simulink model "ME425QuadcoptorMotionControlV2"  (R2024b)
settings: Solver=VariableStepAuto  StartTime=0.0  StopTime=simTime  FixedStep=0.0001  RelTol=1e-2
undefined symbols (not defined in the file): D_phi, D_psi, D_theta, D_z, g, I_phi, I_psi, I_theta, I_z, initialAngles, Ix, Iy, Iz, m, P__phi, P_psi, P_theta, P_z, zDesired
settings Model: Creator=Arda Gencer  LastModifiedBy=Arda Gencer

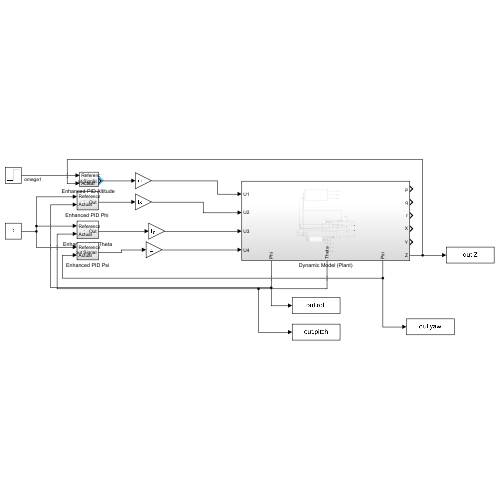
[thumbnail: Simulink's stored preview of the top-level diagram]
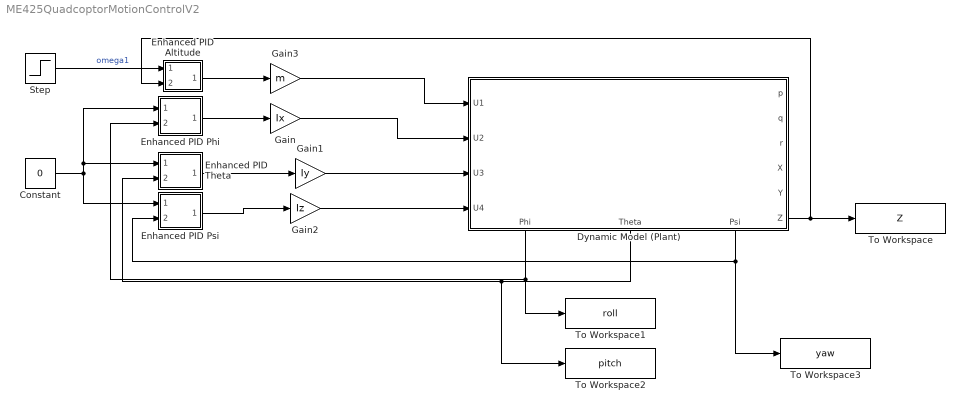
== system ME425QuadcoptorMotionControlV2 ==
  Constant : Constant  Value=0
  Dynamic Model (Plant) : Subsystem
      settings: PortSchema="{\"entries\":[{\"content\":{\"sides\":[{\"content\":{\"connectorIds\":[\"In1\",\"In2\",\"In3\",\"In4\"]},\"type\":\"ConnectorPlacement.EquallySpacedRectSide\",\"uuid\":\"08b1677c-733e-4bff-a275-c4be774b24b5\"},{\"content\":{\"connectorIds\":[\"Out1\",\"Out2\",\"Out3\",\"Out4\",\"Out5\",\"Out6\"],\"side\":\"RIGHT\"},\"type\":\"ConnectorPlacement.EquallySpacedRectSide\",\"uuid\":\"655169e1-9348-4dc0-9050-0d096e576661\"},{\"content\":{\"side\":\"TOP\"},\"type\":\"ConnectorPlacement.EquallySpacedRectSide\",\"uuid\":\"6c01dbd3-88d9-43d1-9966-b2f3dc36f972\"},{\"content\":{\"connectorIds\":[\"Out7\",\"Out8\",\"Out9\"],\"side\":\"BOTTOM\"},\"type\":\"ConnectorPlacement.EquallySpacedRectSide\",\"uuid\":\"d00d5ad9-d72f-434d-885b-77b5f35ca427\"}]},\"type\":\"ConnectorPlacement.EquallySpacedConnector\",\"uuid\":\"87e83324-135b-4426-b2c1-a0cfdb552e41\"}],\"packageUris\":[\"http://schema.mathworks.com/mf0/Connector/R2020b\"],\"version\":\"1.0\"}"
  "Enhanced PID Altitude " : Subsystem
  "Enhanced PID Phi " : Subsystem
  Enhanced PID Psi : Subsystem
  Enhanced PID Theta : Subsystem
  Gain : Gain  Gain=Ix
  Gain1 : Gain  Gain=Iy
  Gain2 : Gain  Gain=Iz
  Gain3 : Gain  Gain=m
  Step : Step  Time=0  After=zDesired  SampleTime=0
  To Workspace : ToWorkspace  VariableName=Z  SampleTime=-1
  To Workspace1 : ToWorkspace  VariableName=roll  SampleTime=-1
  To Workspace2 : ToWorkspace  VariableName=pitch  SampleTime=-1
  To Workspace3 : ToWorkspace  VariableName=yaw  SampleTime=-1
  wires:
  "Enhanced PID Phi "/1(Out) -> Gain/1
  Gain/1 -> Dynamic Model (Plant)/2(U2)
  Gain1/1 -> Dynamic Model (Plant)/3(U3)
  Enhanced PID Theta/1(Out) -> Gain1/1
  Enhanced PID Psi/1(Output Signal) -> Gain2/1
  Gain2/1 -> Dynamic Model (Plant)/4(U4)
  "Enhanced PID Altitude "/1(Output Signal) -> Gain3/1
  Gain3/1 -> Dynamic Model (Plant)/1(U1)
  Dynamic Model (Plant)/6(Z) -> "Enhanced PID Altitude "/2(Actual), To Workspace/1
  Dynamic Model (Plant)/7(Phi) -> To Workspace1/1, "Enhanced PID Phi "/2(Actual)
  Dynamic Model (Plant)/8(Theta) -> To Workspace2/1, Enhanced PID Theta/2(Actual)
  Dynamic Model (Plant)/9(Psi) -> To Workspace3/1, Enhanced PID Psi/2(Actual)
  Constant/1 -> Enhanced PID Psi/1(Reference), Enhanced PID Theta/1(Reference), "Enhanced PID Phi "/1(Reference)
  Step/1 -> "Enhanced PID Altitude "/1(Reference)  "omega1"

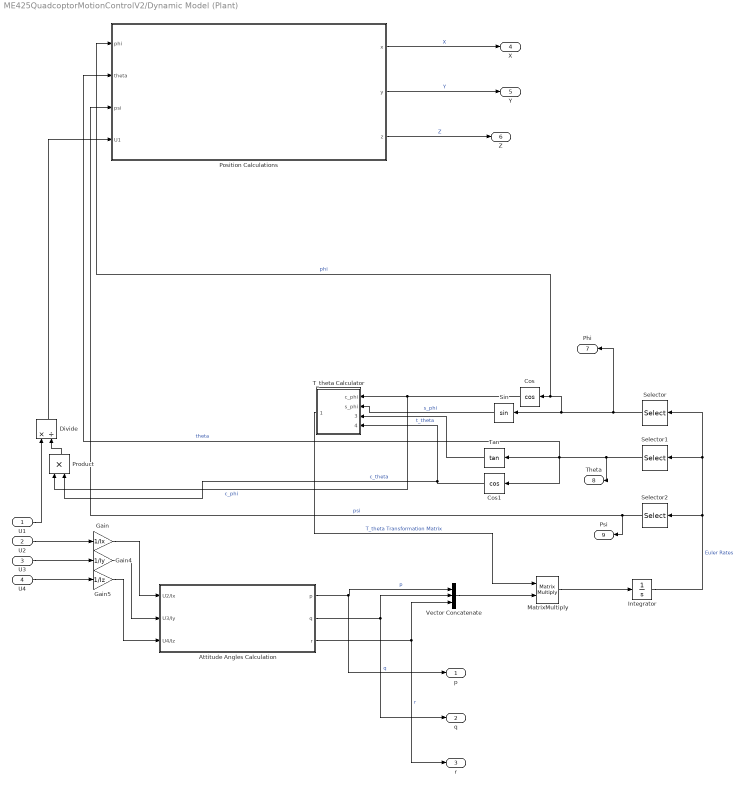
== system ME425QuadcoptorMotionControlV2/Dynamic Model (Plant) ==
  U1 : Inport
  U2 : Inport  Port=2
  U3 : Inport  Port=3
  U4 : Inport  Port=4
  Attitude Angles Calculation : Subsystem
  Cos : Trigonometry  Operator=cos
  Cos1 : Trigonometry  Operator=cos
  Divide : Product  Inputs=*/
  Gain : Gain  Gain=1/Ix
  Gain4 : Gain  Gain=1/Iy
  Gain5 : Gain  Gain=1/Iz
  Integrator : Integrator  InitialCondition=initialAngles
  MatrixMultiply : Product  Multiplication=Matrix(*)
  Position Calculations : Subsystem
  Product : Product
  Selector : Selector  InputPortWidth=3  IndexOptions=Index vector (dialog)  Indices=[1]  OutputSizes=1
  Selector1 : Selector  InputPortWidth=3  IndexOptions=Index vector (dialog)  Indices=2  OutputSizes=1
  Selector2 : Selector  InputPortWidth=3  IndexOptions=Index vector (dialog)  Indices=3  OutputSizes=1
  Sin : Trigonometry
  T_theta Calculator : Subsystem
  Tan : Trigonometry  Operator=tan
  Vector Concatenate : Concatenate  NumInputs=3
  p : Outport
  q : Outport  Port=2
  r : Outport  Port=3
  X : Outport  Port=4
  Y : Outport  Port=5
  Z : Outport  Port=6
  Phi : Outport  Port=7
  Theta : Outport  Port=8
  Psi : Outport  Port=9
  wires:
  Vector Concatenate/1 -> MatrixMultiply/2
  Selector1/1 -> Theta/1, Cos1/1, Position Calculations/2(theta), Tan/1  "theta"
  Attitude Angles Calculation/2(q) -> q/1, Vector Concatenate/2  "q"
  U4/1 -> Gain5/1
  Cos/1 -> Product/1, T_theta Calculator/1(c_phi)  "c_phi"
  Selector/1 -> Phi/1, Position Calculations/1(phi), Cos/1, Sin/1  "phi"
  Gain/1 -> Attitude Angles Calculation/1(U2/Ix)
  Gain5/1 -> Attitude Angles Calculation/3(U4/Iz)
  Attitude Angles Calculation/3(r) -> r/1, Vector Concatenate/3  "r"
  Tan/1 -> T_theta Calculator/3(t_theta)  "t_theta"
  Sin/1 -> T_theta Calculator/2(s_phi)  "s_phi"
  Cos1/1 -> Product/2, T_theta Calculator/4(c_theta)  "c_theta"
  MatrixMultiply/1 -> Integrator/1
  T_theta Calculator/1(T_theta) -> MatrixMultiply/1  "T_theta Transformation Matrix"
  U2/1 -> Gain/1
  U3/1 -> Gain4/1
  Selector2/1 -> Psi/1, Position Calculations/3(psi)  "psi"
  Attitude Angles Calculation/1(p) -> p/1, Vector Concatenate/1  "p"
  Position Calculations/3(z) -> Z/1  "Z"
  Gain4/1 -> Attitude Angles Calculation/2(U3/Iy)
  Position Calculations/1(x) -> X/1  "X"
  Position Calculations/2(y) -> Y/1  "Y"
  U1/1 -> Divide/1
  Divide/1 -> Position Calculations/4(U1)
  Product/1 -> Divide/2
  Integrator/1 -> Selector/1, Selector1/1, Selector2/1  "Euler Rates"

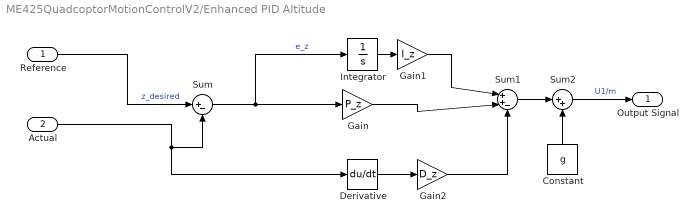
== system ME425QuadcoptorMotionControlV2/Enhanced PID Altitude  ==
  Reference : Inport
  Actual : Inport  Port=2
  Constant : Constant  Value=g
  Derivative : Derivative
  Gain : Gain  Gain=P_z
  Gain1 : Gain  Gain=I_z
  Gain2 : Gain  Gain=D_z
  Integrator : Integrator
  Sum : Sum  Inputs=|+-
  Sum1 : Sum  Inputs=|++-
  Sum2 : Sum  Inputs=|++
  Output Signal : Outport
  wires:
  Actual/1 -> Derivative/1, Sum/2
  Reference/1 -> Sum/1  "z_desired"
  Sum/1 -> Integrator/1, Gain/1  "e_z"
  Derivative/1 -> Gain2/1
  Gain/1 -> Sum1/2
  Integrator/1 -> Gain1/1
  Gain1/1 -> Sum1/1
  Gain2/1 -> Sum1/3
  Sum1/1 -> Sum2/1
  Constant/1 -> Sum2/2
  Sum2/1 -> Output Signal/1  "U1/m"

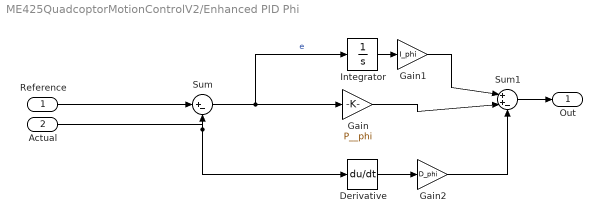
== system ME425QuadcoptorMotionControlV2/Enhanced PID Phi  ==
  Reference : Inport
  Actual : Inport  Port=2
  Derivative : Derivative
  Gain : Gain  Gain=P__phi
  Gain1 : Gain  Gain=I_phi
  Gain2 : Gain  Gain=D_phi
  Integrator : Integrator
  Sum : Sum  Inputs=|+-
  Sum1 : Sum  Inputs=|++-
  Out : Outport
  wires:
  Actual/1 -> Derivative/1, Sum/2
  Reference/1 -> Sum/1
  Sum/1 -> Integrator/1, Gain/1  "e"
  Derivative/1 -> Gain2/1
  Gain/1 -> Sum1/2
  Integrator/1 -> Gain1/1
  Sum1/1 -> Out/1
  Gain1/1 -> Sum1/1
  Gain2/1 -> Sum1/3

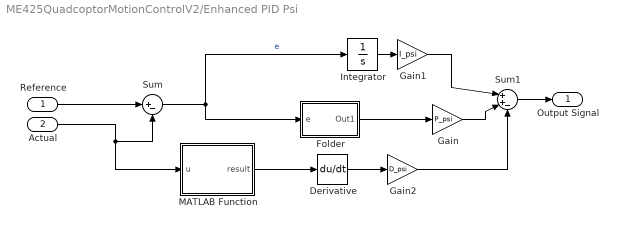
== system ME425QuadcoptorMotionControlV2/Enhanced PID Psi ==
  Reference : Inport
  Actual : Inport  Port=2
  Derivative : Derivative
  Folder : Subsystem
  Gain : Gain  Gain=P_psi
  Gain1 : Gain  Gain=I_psi
  Gain2 : Gain  Gain=D_psi
  Integrator : Integrator
  MATLAB Function : MATLAB Function  TreatAsAtomicUnit=on
  Sum : Sum  Inputs=|+-
  Sum1 : Sum  Inputs=|++-
  Output Signal : Outport
  wires:
  Actual/1 -> MATLAB Function/1(u), Sum/2
  Reference/1 -> Sum/1
  Sum/1 -> Integrator/1, Folder/1(e)  "e"
  Derivative/1 -> Gain2/1
  Gain/1 -> Sum1/2
  Integrator/1 -> Gain1/1
  Sum1/1 -> Output Signal/1
  Gain1/1 -> Sum1/1
  Gain2/1 -> Sum1/3
  Folder/1(Out1) -> Gain/1
  MATLAB Function/1(result) -> Derivative/1

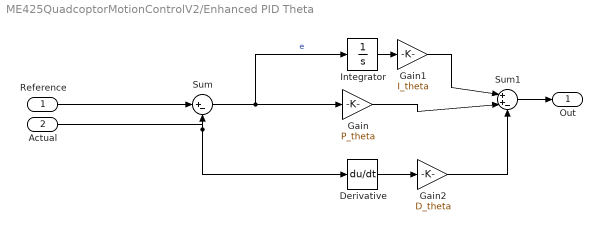
== system ME425QuadcoptorMotionControlV2/Enhanced PID Theta ==
  Reference : Inport
  Actual : Inport  Port=2
  Derivative : Derivative
  Gain : Gain  Gain=P_theta
  Gain1 : Gain  Gain=I_theta
  Gain2 : Gain  Gain=D_theta
  Integrator : Integrator
  Sum : Sum  Inputs=|+-
  Sum1 : Sum  Inputs=|++-
  Out : Outport
  wires:
  Actual/1 -> Derivative/1, Sum/2
  Reference/1 -> Sum/1
  Sum/1 -> Integrator/1, Gain/1  "e"
  Derivative/1 -> Gain2/1
  Gain/1 -> Sum1/2
  Integrator/1 -> Gain1/1
  Sum1/1 -> Out/1
  Gain1/1 -> Sum1/1
  Gain2/1 -> Sum1/3

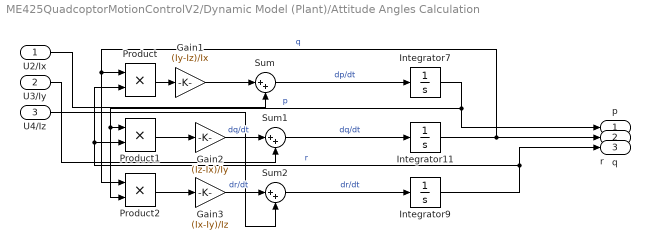
== system ME425QuadcoptorMotionControlV2/Dynamic Model (Plant)/Attitude Angles Calculation ==
  U2/Ix : Inport
  U3/Iy : Inport  Port=2
  U4/Iz : Inport  Port=3
  Gain1 : Gain  Gain=(Iy-Iz)/Ix
  Gain2 : Gain  Gain=(Iz-Ix)/Iy
  Gain3 : Gain  Gain=(Ix-Iy)/Iz
  Integrator11 : Integrator
  Integrator7 : Integrator
  Integrator9 : Integrator
  Product : Product
  Product1 : Product
  Product2 : Product
  Sum : Sum  Inputs=|++
  Sum1 : Sum  Inputs=|++
  Sum2 : Sum  Inputs=|++
  p : Outport
  q : Outport  Port=2
  r : Outport  Port=3
  wires:
  Integrator11/1 -> q/1, Product2/1, Product/1  "q"
  Integrator7/1 -> p/1, Product2/2, Product1/1  "p"
  Gain1/1 -> Sum/1
  Integrator9/1 -> r/1, Product1/2, Product/2  "r"
  Product2/1 -> Gain3/1
  Sum/1 -> Integrator7/1  "dp/dt"
  Product1/1 -> Gain2/1
  Gain2/1 -> Sum1/1  "dq/dt"
  Gain3/1 -> Sum2/1  "dr/dt"
  Sum1/1 -> Integrator11/1  "dq/dt"
  Sum2/1 -> Integrator9/1  "dr/dt"
  U3/Iy/1 -> Sum1/2
  Product/1 -> Gain1/1
  U2/Ix/1 -> Sum/2
  U4/Iz/1 -> Sum2/2

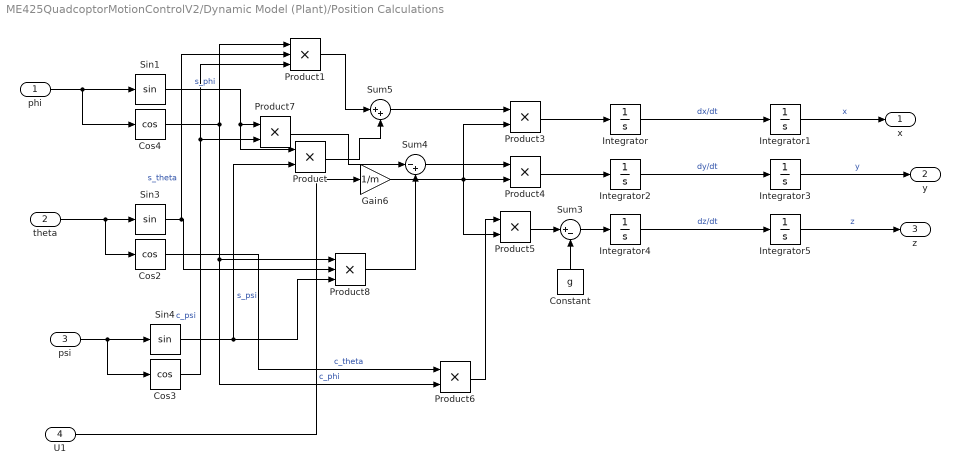
== system ME425QuadcoptorMotionControlV2/Dynamic Model (Plant)/Position Calculations ==
  phi : Inport
  theta : Inport  Port=2
  psi : Inport  Port=3
  U1 : Inport  Port=4
  Constant : Constant  Value=g
  Cos2 : Trigonometry  Operator=cos
  Cos3 : Trigonometry  Operator=cos
  Cos4 : Trigonometry  Operator=cos
  Gain6 : Gain  Gain=1/m
  Integrator{,1..5} (6 alike) : Integrator
  Product{,3..7} (6 alike) : Product
  Product1 : Product  Inputs=3
  Product8 : Product  Inputs=3
  Sin1 : Trigonometry
  Sin3 : Trigonometry
  Sin4 : Trigonometry
  Sum3 : Sum  Inputs=|+-
  Sum4 : Sum  Inputs=|-+
  Sum5 : Sum  Inputs=|++
  x : Outport
  y : Outport  Port=2
  z : Outport  Port=3
  wires:
  Integrator4/1 -> Integrator5/1  "dz/dt"
  Sin3/1 -> Product1/2, Product8/2  "s_theta"
  psi/1 -> Cos3/1, Sin4/1
  U1/1 -> Gain6/1
  Sum4/1 -> Product4/1
  Integrator2/1 -> Integrator3/1  "dy/dt"
  Cos4/1 -> Product8/1, Product6/2, Product1/1  "c_phi"
  Integrator1/1 -> x/1  "x"
  theta/1 -> Cos2/1, Sin3/1
  Gain6/1 -> Product3/2, Product5/2, Product4/2
  Sum3/1 -> Integrator4/1
  Sin4/1 -> Product/2, Product8/3  "s_psi"
  Product1/1 -> Sum5/1
  Integrator/1 -> Integrator1/1  "dx/dt"
  Sum5/1 -> Product3/1
  Cos3/1 -> Product1/3, Product7/2  "c_psi"
  Product3/1 -> Integrator/1
  Product4/1 -> Integrator2/1
  Cos2/1 -> Product6/1  "c_theta"
  phi/1 -> Cos4/1, Sin1/1
  Product7/1 -> Sum4/1
  Product6/1 -> Product5/1
  Product/1 -> Sum5/2
  Constant/1 -> Sum3/2
  Product5/1 -> Sum3/1
  Sin1/1 -> Product/1, Product7/1  "s_phi"
  Product8/1 -> Sum4/2
  Integrator3/1 -> y/1  "y"
  Integrator5/1 -> z/1  "z"

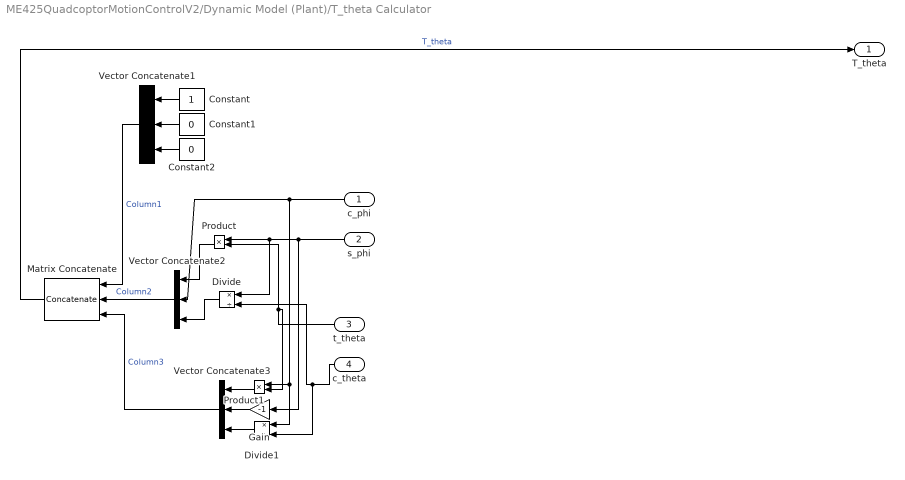
== system ME425QuadcoptorMotionControlV2/Dynamic Model (Plant)/T_theta Calculator ==
  c_phi : Inport
  s_phi : Inport  Port=2
  t_theta : Inport  Port=3
  c_theta : Inport  Port=4
  Constant : Constant
  Constant1 : Constant  Value=0
  Constant2 : Constant  Value=0
  Divide : Product  Inputs=*/
  Divide1 : Product  Inputs=*/
  Gain : Gain  Gain=-1
  Matrix Concatenate : Concatenate  NumInputs=3  Mode=Multidimensional array  ConcatenateDimension=2
  Product : Product
  Product1 : Product
  Vector Concatenate1 : Concatenate  NumInputs=3
  Vector Concatenate2 : Concatenate  NumInputs=3
  Vector Concatenate3 : Concatenate  NumInputs=3
  T_theta : Outport
  wires:
  c_theta/1 -> Divide/2, Divide1/2
  c_phi/1 -> Vector Concatenate2/2, Divide1/1, Product1/1
  Constant/1 -> Vector Concatenate1/1
  Vector Concatenate2/1 -> Matrix Concatenate/2  "Column2"
  Product/1 -> Vector Concatenate2/1
  s_phi/1 -> Product/1, Divide/1, Gain/1
  Product1/1 -> Vector Concatenate3/1
  Vector Concatenate3/1 -> Matrix Concatenate/3  "Column3"
  Matrix Concatenate/1 -> T_theta/1  "T_theta"
  Constant2/1 -> Vector Concatenate1/3
  Constant1/1 -> Vector Concatenate1/2
  Vector Concatenate1/1 -> Matrix Concatenate/1  "Column1"
  t_theta/1 -> Product1/2, Product/2
  Gain/1 -> Vector Concatenate3/2
  Divide1/1 -> Vector Concatenate3/3
  Divide/1 -> Vector Concatenate2/3

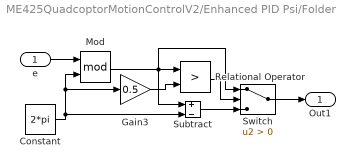
== system ME425QuadcoptorMotionControlV2/Enhanced PID Psi/Folder ==
  e : Inport
  Constant : Constant  Value=2*pi
  Gain3 : Gain  Gain=0.5
  Mod : Math  Operator=mod
  Relational Operator : RelationalOperator  Operator=>  OutDataTypeStr=boolean  RndMeth=Simplest  InputSameDT=off
  Subtract : Sum  Inputs=+-
  Switch : Switch  Criteria=u2 > Threshold  SaturateOnIntegerOverflow=off  InputSameDT=off
  Out1 : Outport
  wires:
  Mod/1 -> Subtract/1, Switch/1, Relational Operator/1
  e/1 -> Mod/1
  Subtract/1 -> Switch/3
  Switch/1 -> Out1/1
  Relational Operator/1 -> Switch/2
  Gain3/1 -> Relational Operator/2
  Constant/1 -> Gain3/1, Mod/2, Subtract/2

== matlab function ME425QuadcoptorMotionControlV2/Enhanced PID Psi/MATLAB Function ==
  settings: updateMethod=DISCRETE  sampleTime=0.001
  data: result output; u input
function result = signCoherence(u)
persistent u_old;
if isempty(u_old)
    u_old = 0;
end

delta = u - u_old;

if delta > pi
    delta = delta - 2*pi;
elseif delta < -pi
    delta = delta + 2*pi;
end

u_old = u;
result = delta;
end
